simulink model "mass_spring_damper"  (R2016a)
settings: Solver=VariableStepAuto  StartTime=0.0  StopTime=20  MaxStep=1e-2  RelTol=1e-3
values from neighbouring files (symbols this model uses):
  b = 1    [E10.m]    (also in E10b.m; E11.m = 4; E12.m = 0.5; E13.m = 0.5)
  F = 5    [E10.m]    (also in E10b.m; E11.m; E12.m; E13.m)
  k = 1    [E10.m]    (also in E10b.m; E11.m; E12.m; E13.m)
  m = 1    [E10.m]    (also in E10b.m; E11.m; E12.m; E13.m)
settings Model: Creator=alepen  LastModifiedBy=alepen
settings DataIOCC: SaveFormat=StructureWithTime  StreamToWorkspace=on

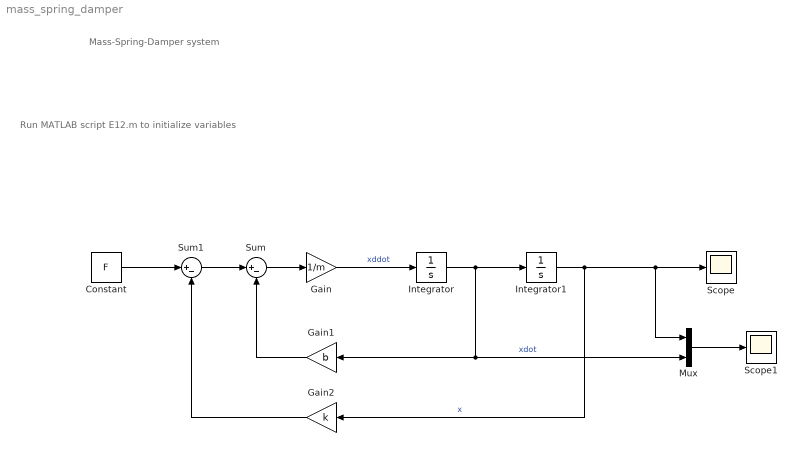
== system mass_spring_damper ==
  note: Run MATLAB script E12.m to initialize variables
  note: Mass-Spring-Damper system
  Constant : Constant  Value=F
  Gain : Gain  Gain=1/m
  Gain1 : Gain  Gain=b
  Gain2 : Gain  Gain=k
  Integrator : Integrator
  Integrator1 : Integrator
  Mux : Mux  Inputs=2
  Scope : Scope
  Scope1 : Scope
  Sum : Sum  Inputs=|+-
  Sum1 : Sum  Inputs=|+-
  wires:
  Integrator/1 -> Mux/2, Gain1/1, Integrator1/1  "xdot"
  Sum/1 -> Gain/1
  Integrator1/1 -> Gain2/1, Mux/1, Scope/1  "x"
  Gain/1 -> Integrator/1  "xddot"
  Sum1/1 -> Sum/1
  Constant/1 -> Sum1/1
  Gain1/1 -> Sum/2
  Gain2/1 -> Sum1/2
  Mux/1 -> Scope1/1
